simulink model "c6701evmDIPswitch"  (Simulink 6.0)
settings: Solver=FixedStepDiscrete  StartTime=0.0  StopTime=inf  RelTol=1e-3
libraries: c6701evmlib x4, dspsigops x4, c6000tgtpreflib x1
settings Model: Creator=zgalijas  LastModifiedBy=thartley  RTWExpressionDepthLimit=1  ProdHWDeviceType=TI C6000
settings DataIOCC: LimitDataPoints=off  SaveOutput=off  SaveTime=off  SignalLoggingName=sigsOut
settings OptimizationCC: InlineParams=on  InlineInvariantSignals=off  EnforceIntegerDowncast=off
settings DebuggingCC: CheckExecutionContextPreStartOutputMsg=on  CheckExecutionContextRuntimeOutputMsg=on  SolverPrmCheckMsg=none
settings HardwareCC: ProdBitPerLong=40  ProdEndianess=LittleEndian  ProdHWDeviceType=TI C6000
settings ModelReferenceCC: UpdateModelReferenceTargets=IfOutOfDate
settings RTWCC: SystemTargetFile=ti_c6000.tlc  TemplateMakefile=ti_c6000.tmf  ProcessScript=ti_c6000_make_rtw_hook
settings CodeAppCC: PrefixModelToSubsysFcnNames=off
settings STFCustomTargetCC: TargetFcnLib=ansi_tfl_tmw.mat  MatFileLogging=on  LifeSpan=inf  SystemTargetFile=ti_c6000.tlc  ActivateCallback=c6000_callback('ActivateCallback',hSrc,hDlg);
settings GRTTargetCC: ModelReferenceCompliant=off  LifeSpan=inf
settings CustomProperty: DataType=RTWOptions_EnumType_S__A_matlab_toolbox_rtw_targets_tic6000_tic6000_ti_c6000_BoardType  Value=C6701EVM
settings EnumStrPairs: String=C6416DSK
settings SFSimCC: SFSimApplyToAllLibs=on  SFSimBuildMode=Incremental

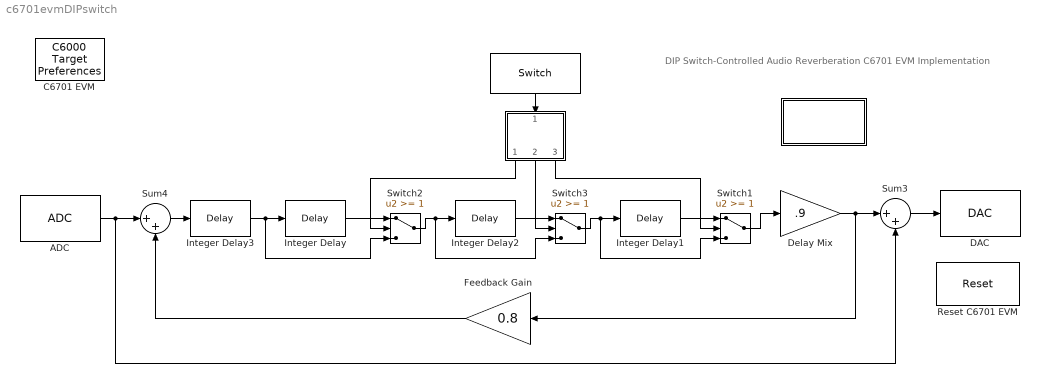
== system c6701evmDIPswitch ==
  note: DIP Switch-Controlled Audio Reverberation
      | C6701 EVM Implementation
  " " : Subsystem
      mask Display: disp('Info')
  "  " : Subsystem  Orientation=down
  "   " : c6701evmlib/Switch  Orientation=down  sw1=off  sw2=off  sw3=off  dType=Boolean  Ts=64/8000
  ADC : c6701evmlib/ADC  ADCsource=Mic In  MicGain=on  Stereo=off  SampleRate=8000  CodecDataFormat=16-bit linear  OutputDataType=Double  Scaling=Normalize  SourceGain=4.5  FrameSize=64
  C6701 EVM : c6000tgtpreflib/C6000 Target Preferences
  DAC : c6701evmlib/DAC  CodecDataFormat=16-bit linear  Scaling=Normalize  DacAtten=0.0  OverflowMode=Saturate
  Delay Mix : Gain  Gain=.9  SaturateOnIntegerOverflow=on
  Feedback Gain : Gain  Orientation=left  Gain=0.8  SaturateOnIntegerOverflow=on
  Integer Delay{,1..3} (4 alike) : dspsigops/Delay  dly_unit=Samples  delay=450  ic_detail=off  dif_ic_for_ch=off  dif_ic_for_dly=off  ic=0  reset_popup=None
  Reset C6701 EVM : c6701evmlib/Reset
  Sum3 : Sum  Inputs=|++  SaturateOnIntegerOverflow=on  InputSameDT=on
  Sum4 : Sum  Inputs=|++  SaturateOnIntegerOverflow=on  InputSameDT=on
  Switch1 : Switch  Threshold=1  ZeroCross=off  InputSameDT=on
  Switch2 : Switch  Threshold=1  ZeroCross=off  InputSameDT=on
  Switch3 : Switch  Threshold=1  ZeroCross=off  InputSameDT=on
  wires:
  Sum3/1 -> DAC/1
  ADC/1 -> Sum3/2, Sum4/1
  Feedback Gain/1 -> Sum4/2
  Delay Mix/1 -> Feedback Gain/1, Sum3/1
  Switch1/1 -> Delay Mix/1
  Integer Delay1/1 -> Switch1/1
  Integer Delay/1 -> Switch2/1
  Switch2/1 -> Integer Delay2/1, Switch3/3
  "  "/1(SW0) -> Switch2/2
  Sum4/1 -> Integer Delay3/1
  Integer Delay3/1 -> Integer Delay/1, Switch2/3
  Integer Delay2/1 -> Switch3/1
  Switch3/1 -> Integer Delay1/1, Switch1/3
  "  "/2(SW1) -> Switch3/2
  "  "/3(SW2) -> Switch1/2
  "   "/1 -> "  "/1("   ")

== system c6701evmDIPswitch/  ==
  note: DIP Switch-Controlled Audio Reverberation
      | C6701 EVM Implementation
      |
      | This simulation of audio reverberation demonstrates the use of the C6701 EVM DIP Switch block.
      | This block reads the status of user-controlled DIP switches (USER0, USER1, USER2) on
      | the c6701 EVM board. Each DIP switch controls a corresponding delay block.

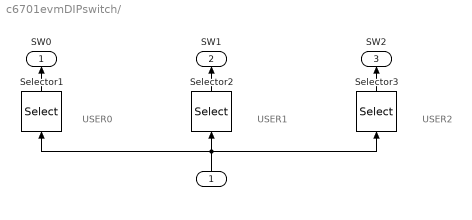
== system c6701evmDIPswitch/   ==
  note: USER0
  note: USER1
  note: USER2
  "   " : Inport  Orientation=up
  Selector1 : Selector  Orientation=up  InputPortWidth=3
  Selector2 : Selector  Orientation=up  Elements=2  InputPortWidth=3
  Selector3 : Selector  Orientation=up  Elements=3  InputPortWidth=3
  SW0 : Outport  Orientation=up
  SW1 : Outport  Orientation=up  Port=2
  SW2 : Outport  Orientation=up  Port=3
  wires:
  "   "/1 -> Selector2/1, Selector3/1, Selector1/1
  Selector1/1 -> SW0/1
  Selector2/1 -> SW1/1
  Selector3/1 -> SW2/1
